simulink model "multi_agent_SVFB"  (R2023a)
settings: Solver=VariableStepAuto  StartTime=0.0  StopTime=t_sim  RelTol=1e-3
values from neighbouring files (symbols this model uses):
  A = A_contr    [e03_main.m]
  A0 = A    [e03_main.m]
  Adj = zeros(6,6)    [e03_main.m]
  B = [ ... (first row only)    [e03_main.m]
  C = eye(4)    [e03_main.m]
  c = 2*c_min    [e03_main.m]
  D = zeros(4,1)    [e03_main.m]
  g = zeros(6,1)    [e03_main.m]
  K = inv(R)*B'*P    [e03_main.m]
  K_contr = place(A,B, 0.5*[0 -1 -2 -3])    [e03_main.m]
  x0_0 = [10 0 0 0]    [e03_main.m]
  xi_0 = zeros(4,1)    [e03_main.m]
settings Model: Creator=federico  LastModifiedBy=federico

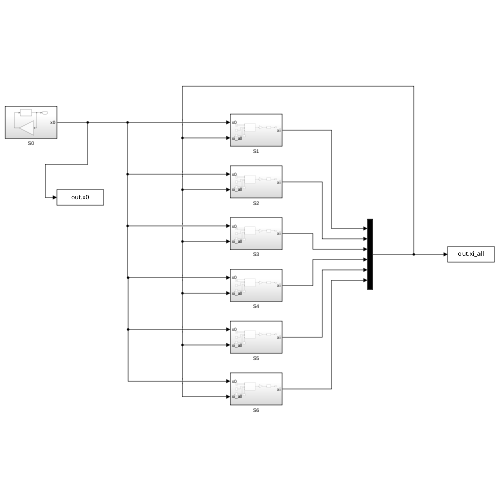
[thumbnail: Simulink's stored preview of the top-level diagram]
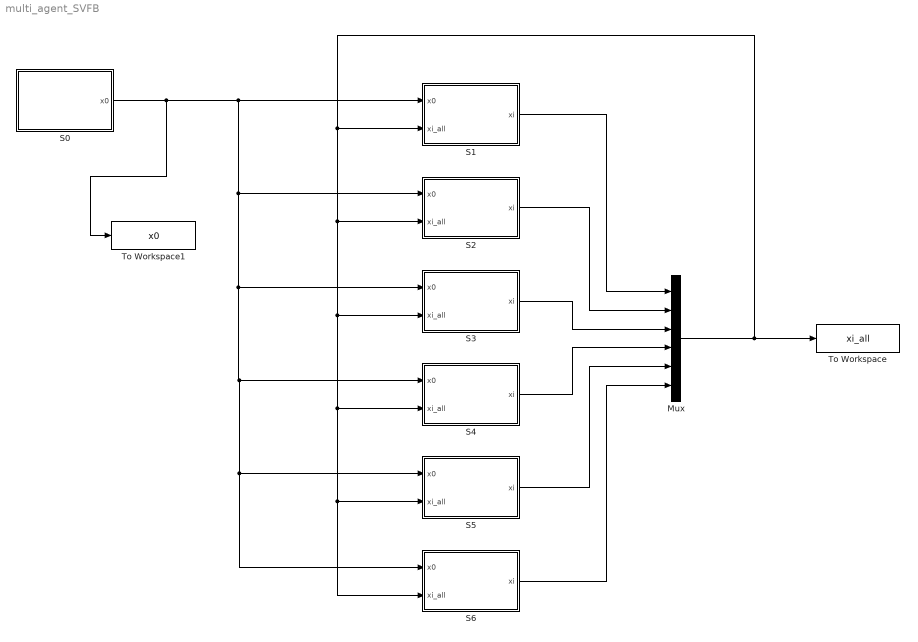
== system multi_agent_SVFB ==
  Mux : Mux  Inputs=6
  S0 : Subsystem
  S1 : Subsystem
  S2 : Subsystem
  S3 : Subsystem
  S4 : Subsystem
  S5 : Subsystem
  S6 : Subsystem
  To Workspace : ToWorkspace  VariableName=xi_all  SampleTime=-1
  To Workspace1 : ToWorkspace  VariableName=x0  SampleTime=-1
  wires:
  S1/1(xi) -> Mux/1
  S2/1(xi) -> Mux/2
  S3/1(xi) -> Mux/3
  S4/1(xi) -> Mux/4
  S5/1(xi) -> Mux/5
  S6/1(xi) -> Mux/6
  Mux/1 -> To Workspace/1, S6/2(xi_all), S5/2(xi_all), S4/2(xi_all), S3/2(xi_all), S2/2(xi_all), S1/2(xi_all)
  S0/1(x0) -> To Workspace1/1, S6/1(x0), S5/1(x0), S4/1(x0), S3/1(x0), S2/1(x0), S1/1(x0)

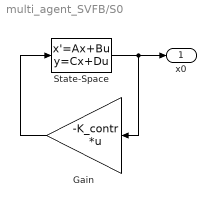
== system multi_agent_SVFB/S0 ==
  Gain : Gain  Gain=-K_contr  Multiplication=Matrix(K*u)
  State-Space : StateSpace  A=A0  B=B  C=C  D=D  InitialCondition=x0_0
  x0 : Outport
  wires:
  State-Space/1 -> Gain/1, x0/1
  Gain/1 -> State-Space/1

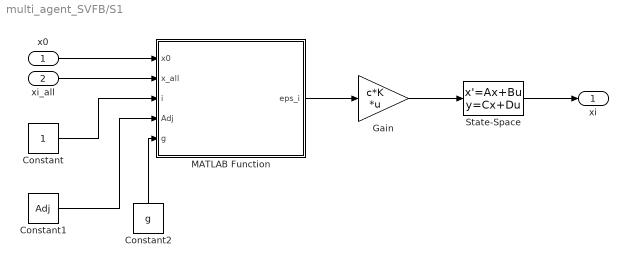
== system multi_agent_SVFB/S1 ==
  x0 : Inport
  xi_all : Inport  Port=2
  Constant : Constant
  Constant1 : Constant  Value=Adj
  Constant2 : Constant  Value=g
  Gain : Gain  Gain=c*K  Multiplication=Matrix(K*u)
  MATLAB Function : MATLAB Function  TreatAsAtomicUnit=on
  State-Space : StateSpace  A=A  B=B  C=C  D=D  InitialCondition=xi_0
  xi : Outport
  wires:
  State-Space/1 -> xi/1
  Gain/1 -> State-Space/1
  MATLAB Function/1(eps_i) -> Gain/1
  x0/1 -> MATLAB Function/1(x0)
  xi_all/1 -> MATLAB Function/2(x_all)
  Constant/1 -> MATLAB Function/3(i)
  Constant1/1 -> MATLAB Function/4(Adj)
  Constant2/1 -> MATLAB Function/5(g)

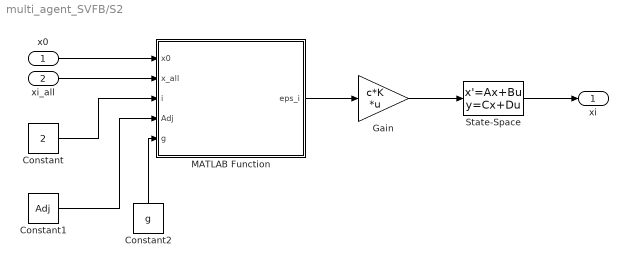
== system multi_agent_SVFB/S2 ==
  x0 : Inport
  xi_all : Inport  Port=2
  Constant : Constant  Value=2
  Constant1 : Constant  Value=Adj
  Constant2 : Constant  Value=g
  Gain : Gain  Gain=c*K  Multiplication=Matrix(K*u)
  MATLAB Function : MATLAB Function  TreatAsAtomicUnit=on
  State-Space : StateSpace  A=A  B=B  C=C  D=D  InitialCondition=xi_0
  xi : Outport
  wires:
  State-Space/1 -> xi/1
  Gain/1 -> State-Space/1
  MATLAB Function/1(eps_i) -> Gain/1
  x0/1 -> MATLAB Function/1(x0)
  xi_all/1 -> MATLAB Function/2(x_all)
  Constant/1 -> MATLAB Function/3(i)
  Constant1/1 -> MATLAB Function/4(Adj)
  Constant2/1 -> MATLAB Function/5(g)

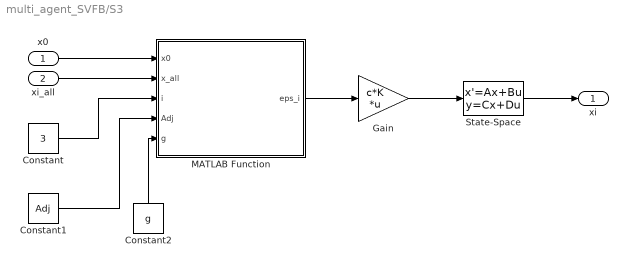
== system multi_agent_SVFB/S3 ==
  x0 : Inport
  xi_all : Inport  Port=2
  Constant : Constant  Value=3
  Constant1 : Constant  Value=Adj
  Constant2 : Constant  Value=g
  Gain : Gain  Gain=c*K  Multiplication=Matrix(K*u)
  MATLAB Function : MATLAB Function  TreatAsAtomicUnit=on
  State-Space : StateSpace  A=A  B=B  C=C  D=D  InitialCondition=xi_0
  xi : Outport
  wires:
  State-Space/1 -> xi/1
  Gain/1 -> State-Space/1
  MATLAB Function/1(eps_i) -> Gain/1
  x0/1 -> MATLAB Function/1(x0)
  xi_all/1 -> MATLAB Function/2(x_all)
  Constant/1 -> MATLAB Function/3(i)
  Constant1/1 -> MATLAB Function/4(Adj)
  Constant2/1 -> MATLAB Function/5(g)

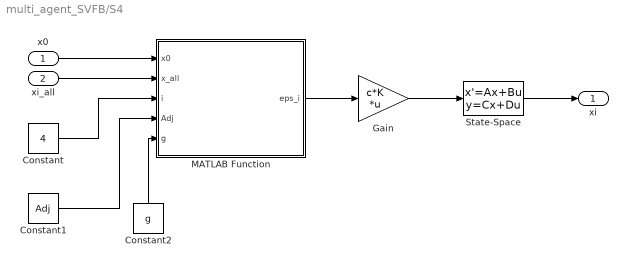
== system multi_agent_SVFB/S4 ==
  x0 : Inport
  xi_all : Inport  Port=2
  Constant : Constant  Value=4
  Constant1 : Constant  Value=Adj
  Constant2 : Constant  Value=g
  Gain : Gain  Gain=c*K  Multiplication=Matrix(K*u)
  MATLAB Function : MATLAB Function  TreatAsAtomicUnit=on
  State-Space : StateSpace  A=A  B=B  C=C  D=D  InitialCondition=xi_0
  xi : Outport
  wires:
  State-Space/1 -> xi/1
  Gain/1 -> State-Space/1
  MATLAB Function/1(eps_i) -> Gain/1
  x0/1 -> MATLAB Function/1(x0)
  xi_all/1 -> MATLAB Function/2(x_all)
  Constant/1 -> MATLAB Function/3(i)
  Constant1/1 -> MATLAB Function/4(Adj)
  Constant2/1 -> MATLAB Function/5(g)

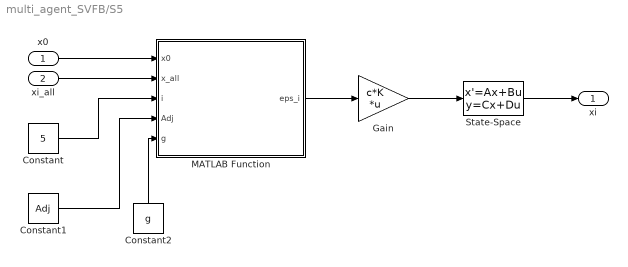
== system multi_agent_SVFB/S5 ==
  x0 : Inport
  xi_all : Inport  Port=2
  Constant : Constant  Value=5
  Constant1 : Constant  Value=Adj
  Constant2 : Constant  Value=g
  Gain : Gain  Gain=c*K  Multiplication=Matrix(K*u)
  MATLAB Function : MATLAB Function  TreatAsAtomicUnit=on
  State-Space : StateSpace  A=A  B=B  C=C  D=D  InitialCondition=xi_0
  xi : Outport
  wires:
  State-Space/1 -> xi/1
  Gain/1 -> State-Space/1
  MATLAB Function/1(eps_i) -> Gain/1
  x0/1 -> MATLAB Function/1(x0)
  xi_all/1 -> MATLAB Function/2(x_all)
  Constant/1 -> MATLAB Function/3(i)
  Constant1/1 -> MATLAB Function/4(Adj)
  Constant2/1 -> MATLAB Function/5(g)

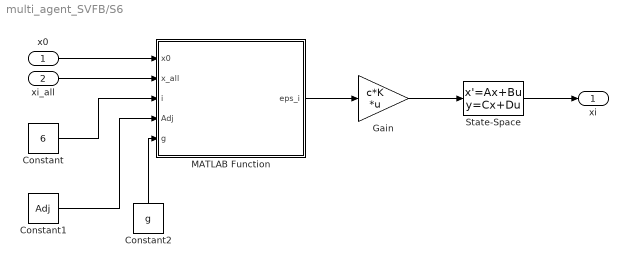
== system multi_agent_SVFB/S6 ==
  x0 : Inport
  xi_all : Inport  Port=2
  Constant : Constant  Value=6
  Constant1 : Constant  Value=Adj
  Constant2 : Constant  Value=g
  Gain : Gain  Gain=c*K  Multiplication=Matrix(K*u)
  MATLAB Function : MATLAB Function  TreatAsAtomicUnit=on
  State-Space : StateSpace  A=A  B=B  C=C  D=D  InitialCondition=xi_0
  xi : Outport
  wires:
  State-Space/1 -> xi/1
  Gain/1 -> State-Space/1
  MATLAB Function/1(eps_i) -> Gain/1
  x0/1 -> MATLAB Function/1(x0)
  xi_all/1 -> MATLAB Function/2(x_all)
  Constant/1 -> MATLAB Function/3(i)
  Constant1/1 -> MATLAB Function/4(Adj)
  Constant2/1 -> MATLAB Function/5(g)

== matlab function multi_agent_SVFB/S2/MATLAB Function ==
  data: x0 input; x_all input; eps_i output; i input; Adj input; g input
function eps_i = fcn(x0, x_all, i, Adj, g)

x_all = reshape(x_all, [4,6]);

eps_i = zeros(4,1);
for j = 1:size(Adj,1)
    eps_i = eps_i + Adj(i,j) * (x_all(:,j) - x_all(:,i));
end
eps_i = eps_i + g(i) * (x0 - x_all(:,i));

== matlab function multi_agent_SVFB/S1/MATLAB Function ==
  data: x0 input; x_all input; eps_i output; i input; Adj input; g input
function eps_i = fcn(x0, x_all, i, Adj, g)

x_all = reshape(x_all, [4,6]);

eps_i = zeros(4,1);
for j = 1:size(Adj,1)
    eps_i = eps_i + Adj(i,j) * (x_all(:,j) - x_all(:,i));
end
eps_i = eps_i + g(i) * (x0 - x_all(:,i));

== matlab function multi_agent_SVFB/S3/MATLAB Function ==
  data: x0 input; x_all input; eps_i output; i input; Adj input; g input
function eps_i = fcn(x0, x_all, i, Adj, g)

x_all = reshape(x_all, [4,6]);

eps_i = zeros(4,1);
for j = 1:size(Adj,1)
    eps_i = eps_i + Adj(i,j) * (x_all(:,j) - x_all(:,i));
end
eps_i = eps_i + g(i) * (x0 - x_all(:,i));

== matlab function multi_agent_SVFB/S4/MATLAB Function ==
  data: x0 input; x_all input; eps_i output; i input; Adj input; g input
function eps_i = fcn(x0, x_all, i, Adj, g)

x_all = reshape(x_all, [4,6]);

eps_i = zeros(4,1);
for j = 1:size(Adj,1)
    eps_i = eps_i + Adj(i,j) * (x_all(:,j) - x_all(:,i));
end
eps_i = eps_i + g(i) * (x0 - x_all(:,i));

== matlab function multi_agent_SVFB/S5/MATLAB Function ==
  data: x0 input; x_all input; eps_i output; i input; Adj input; g input
function eps_i = fcn(x0, x_all, i, Adj, g)

x_all = reshape(x_all, [4,6]);

eps_i = zeros(4,1);
for j = 1:size(Adj,1)
    eps_i = eps_i + Adj(i,j) * (x_all(:,j) - x_all(:,i));
end
eps_i = eps_i + g(i) * (x0 - x_all(:,i));

== matlab function multi_agent_SVFB/S6/MATLAB Function ==
  data: x0 input; x_all input; eps_i output; i input; Adj input; g input
function eps_i = fcn(x0, x_all, i, Adj, g)

x_all = reshape(x_all, [4,6]);

eps_i = zeros(4,1);
for j = 1:size(Adj,1)
    eps_i = eps_i + Adj(i,j) * (x_all(:,j) - x_all(:,i));
end
eps_i = eps_i + g(i) * (x0 - x_all(:,i));
